simulink model "ckl_08022311_8_8"  (R2022b)
settings: Solver=VariableStepAuto  StartTime=0.0  StopTime=100  RelTol=1e-3
settings Model: Creator=ASUS  LastModifiedBy=ASUS

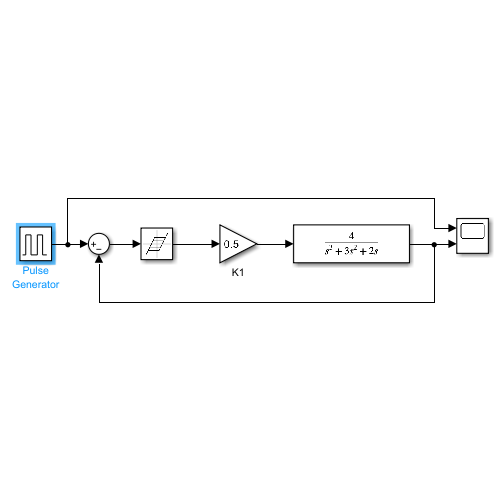
[thumbnail: Simulink's stored preview of the top-level diagram]
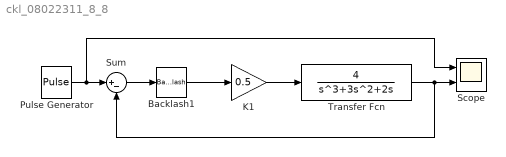
== system ckl_08022311_8_8 ==
  Backlash1 : Backlash  BacklashWidth=2
  K1 : Gain  Gain=0.5
  Pulse Generator : DiscretePulseGenerator  PulseType=Time based  Amplitude=100  Period=100  PulseWidth=0.1
  Scope : Scope  NumInputPorts=2
  Sum : Sum  Inputs=|+-
  Transfer Fcn : TransferFcn  Numerator=[4]  Denominator=[1 3 2 0]
  wires:
  Transfer Fcn/1 -> Scope/2, Sum/2
  Pulse Generator/1 -> Sum/1, Scope/1
  Backlash1/1 -> K1/1
  K1/1 -> Transfer Fcn/1
  Sum/1 -> Backlash1/1
